simulink model "Autopilot"  (R2025a)
settings: Solver=FixedStepDiscrete  StartTime=0.0  StopTime=600  FixedStep=0.008333  RelTol=1e-3
libraries: slpidlib x2
settings Model: Creator=HP  LastModifiedBy=HP
settings DataIOCC: SaveOutput=off  StreamToWks=off  SaveTime=off  ReturnWorkspaceOutputs=off

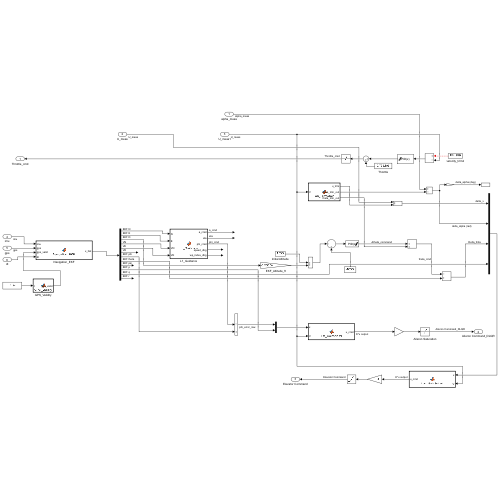
[thumbnail: Simulink's stored preview of the top-level diagram]
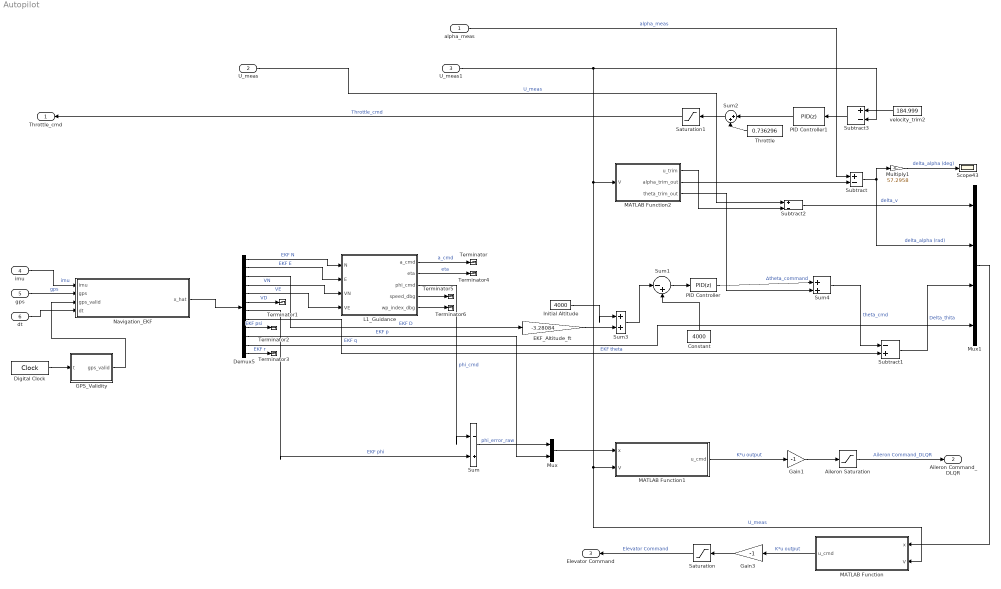
== system Autopilot ==
  alpha_meas : Inport  OutDataTypeStr=double  PortDimensions=1  SampleTime=[0.0083330000000000001,0]
  U_meas : Inport  Port=2  OutDataTypeStr=double  PortDimensions=1  SampleTime=[0.0083330000000000001,0]
  U_meas1 : Inport  Port=3  OutDataTypeStr=double  PortDimensions=1  SampleTime=[0.0083330000000000001,0]
  imu : Inport  Port=4  OutDataTypeStr=double  PortDimensions=[6 1]  SampleTime=[0.0083330000000000001,0]
  gps : Inport  Port=5  OutDataTypeStr=double  PortDimensions=[3 1]  SampleTime=[0.0083330000000000001,0]
  dt : Inport  Port=6  OutDataTypeStr=double  PortDimensions=1  SampleTime=[0.0083330000000000001,0]
  Aileron Saturation : Saturate  UpperLimit=1  LowerLimit=-1
  Constant : Constant  Value=4000  SampleTime=0.008333
  Demux5 : Demux  Outputs=12
  Digital Clock : DigitalClock  SampleTime=0.008333
  EKF_Altitude_ft : Gain  Gain=-3.28084
  GPS_Validity : MATLAB Function  TreatAsAtomicUnit=on  SystemSampleTime=0.008333
  Gain1 : Gain  Gain=-1
  Gain3 : Gain  Gain=-1
  Initial Altitude : Constant  Value=4000  SampleTime=0.008333
  L1_Guidance : MATLAB Function  TreatAsAtomicUnit=on  SystemSampleTime=0.008333
  MATLAB Function : MATLAB Function  TreatAsAtomicUnit=on  SystemSampleTime=0.008333
  MATLAB Function1 : MATLAB Function  TreatAsAtomicUnit=on  SystemSampleTime=0.008333
  MATLAB Function2 : MATLAB Function  TreatAsAtomicUnit=on
  Multiply1 : Gain  Gain=57.2958
  Mux : Mux  Inputs=2
  Mux1 : Mux
  Navigation_EKF : MATLAB Function  TreatAsAtomicUnit=on  SystemSampleTime=0.008333
  PID Controller : slpidlib/PID Controller  Controller=PID  Form=Parallel  TimeDomain=Discrete-time  UseExternalTs=off  SampleTime=0.008333  IntegratorMethod=Forward Euler  FilterMethod=Forward Euler  ControllerParametersSource=internal  P=0.01  I=0.00001  UseKiTs=off  D=0.01  UseExternalDerivativeSource=off  N=115.919945582358  UseFilter=on  TunerSelectOption=Transfer Function Based (PID Tuner App)  InitialConditionSource=internal  InitialConditionForIntegrator=0  InitialConditionForFilter=0  DifferentiatorICPrevScaledInput=0  ExternalReset=none  TrackingMode=off  Kt=1  LimitOutput=on  SatLimitsSource=internal  UpperSaturationLimit=0.2618  LowerSaturationLimit=-0.1745  LinearizeAsGain=on  AntiWindupMode=clamping  Kb=1  LimitIntegrator=off  UpperIntegratorSaturationLimit=inf  LowerIntegratorSaturationLimit=-inf  POutMin=[]  POutMax=[]  IOutMin=[]  IOutMax=[]  DOutMin=[]  DOutMax=[]  NOutMin=[]  NOutMax=[]  SumOutMin=[]  SumOutMax=[]  SaturationOutMin=[]  SaturationOutMax=[]  PParamMin=[]  PParamMax=[]  IParamMin=[]  IParamMax=[]  DParamMin=[]  DParamMax=[]  NParamMin=[]  NParamMax=[]  KbParamMin=[]  KbParamMax=[]  KtParamMin=[]  KtParamMax=[]  KbOutMin=[]  KbOutMax=[]  KtOutMin=[]  KtOutMax=[]  IntegratorOutMin=[]  IntegratorOutMax=[]  FilterOutMin=[]  FilterOutMax=[]  SumI1OutMin=[]  SumI1OutMax=[]  SumI2OutMin=[]  SumI2OutMax=[]  SumI3OutMin=[]  SumI3OutMax=[]  SumI4OutMin=[]  SumI4OutMax=[]  SumDOutMin=[]  SumDOutMax=[]  DifferentiatorOutMin=[]  DifferentiatorOutMax=[]  FilterDiffOutCoefMin=[]  FilterDiffOutCoefMax=[]  ReciprocalOutMin=[]  ReciprocalOutMax=[]  SumDenOutMin=[]  SumDenOutMax=[]  SumNumOutMin=[]  SumNumOutMax=[]  DivideOutMin=[]  DivideOutMax=[]  UdiffTsProdOutMin=[]  UdiffTsProdOutMax=[]  NTsProdOutMin=[]  NTsProdOutMax=[]  UintegralTsProdOutMin=[]  UintegralTsProdOutMax=[]  UngainTsProdOutMin=[]  UngainTsProdOutMax=[]  ClampingZeroOutDataTypeStr=Inherit: Inherit via back propagation  ClampingZeroOutMin=[]  ClampingZeroOutMax=[]  FilterDenConstantOutDataTypeStr=Inherit: Inherit via back propagation  FilterDenConstantOutMin=[]  FilterDenConstantOutMax=[]  PCopyOutDataTypeStr=Inherit: Inherit via back propagation  PCopyOutMin=[]  PCopyOutMax=[]  NCopyOutDataTypeStr=Inherit: Inherit via back propagation  NCopyOutMin=[]  NCopyOutMax=[]  IntegratorContinuousStateAttributes=''  IntegratorStateMustResolveToSignalObject=off  IntegratorRTWStateStorageClass=Auto  FilterContinuousStateAttributes=''  FilterStateMustResolveToSignalObject=off  FilterRTWStateStorageClass=Auto  ParallelPVariant=InternalParameters  IdealPVariant=Disabled  IVariant=InternalParameters  DVariant=InternalParameters  IntegratorVariant=Discrete  SatVariant=Enabled  AWVariant=DiscClampingParallel  PCopyVariant=Disabled  TRVariant=Disabled  FdbkBlocksVariant=Forward  IdealPFdbkVariant=Disabled  SatFdbkVariant=Disabled  DerivativeFilterVariant=ForwardEulerFilter  NVariant=InternalParameters  NCopyVariant=Disabled  FilterICVariant=InternalICsFilter  IntegratorICVariant=InternalICs  ExternalResetVariant=Disabled  TRSumVariant=Passthrough  SumFdbkVariant=Disabled  SumVariant=Sum_PID  TsampFilterVariant=InternalTs  TsampNgainVariant=Passthrough  TsampIntegralVariant=Disabled_SignalSpec  ExternalSaturationOutDataTypeStr=Inherit: Same as second input  DerivativeSourceVariant=ErrorSignal  PreIntVariant=InternalPreInt
  PID Controller1 : slpidlib/PID Controller  Controller=PID  Form=Parallel  TimeDomain=Discrete-time  UseExternalTs=off  SampleTime=0.008333  IntegratorMethod=Forward Euler  FilterMethod=Forward Euler  ControllerParametersSource=internal  P=0.01  I=0.001  UseKiTs=off  D=0  UseExternalDerivativeSource=off  N=100  UseFilter=on  TunerSelectOption=Transfer Function Based (PID Tuner App)  InitialConditionSource=internal  InitialConditionForIntegrator=0  InitialConditionForFilter=0  DifferentiatorICPrevScaledInput=0  ExternalReset=none  TrackingMode=off  Kt=1  LimitOutput=on  SatLimitsSource=internal  UpperSaturationLimit=+0.26  LowerSaturationLimit=-0.73  LinearizeAsGain=on  AntiWindupMode=clamping  Kb=1  LimitIntegrator=off  UpperIntegratorSaturationLimit=inf  LowerIntegratorSaturationLimit=-inf  POutMin=[]  POutMax=[]  IOutMin=[]  IOutMax=[]  DOutMin=[]  DOutMax=[]  NOutMin=[]  NOutMax=[]  SumOutMin=[]  SumOutMax=[]  SaturationOutMin=[]  SaturationOutMax=[]  PParamMin=[]  PParamMax=[]  IParamMin=[]  IParamMax=[]  DParamMin=[]  DParamMax=[]  NParamMin=[]  NParamMax=[]  KbParamMin=[]  KbParamMax=[]  KtParamMin=[]  KtParamMax=[]  KbOutMin=[]  KbOutMax=[]  KtOutMin=[]  KtOutMax=[]  IntegratorOutMin=[]  IntegratorOutMax=[]  FilterOutMin=[]  FilterOutMax=[]  SumI1OutMin=[]  SumI1OutMax=[]  SumI2OutMin=[]  SumI2OutMax=[]  SumI3OutMin=[]  SumI3OutMax=[]  SumI4OutMin=[]  SumI4OutMax=[]  SumDOutMin=[]  SumDOutMax=[]  DifferentiatorOutMin=[]  DifferentiatorOutMax=[]  FilterDiffOutCoefMin=[]  FilterDiffOutCoefMax=[]  ReciprocalOutMin=[]  ReciprocalOutMax=[]  SumDenOutMin=[]  SumDenOutMax=[]  SumNumOutMin=[]  SumNumOutMax=[]  DivideOutMin=[]  DivideOutMax=[]  UdiffTsProdOutMin=[]  UdiffTsProdOutMax=[]  NTsProdOutMin=[]  NTsProdOutMax=[]  UintegralTsProdOutMin=[]  UintegralTsProdOutMax=[]  UngainTsProdOutMin=[]  UngainTsProdOutMax=[]  ClampingZeroOutDataTypeStr=Inherit: Inherit via back propagation  ClampingZeroOutMin=[]  ClampingZeroOutMax=[]  FilterDenConstantOutDataTypeStr=Inherit: Inherit via back propagation  FilterDenConstantOutMin=[]  FilterDenConstantOutMax=[]  PCopyOutDataTypeStr=Inherit: Inherit via back propagation  PCopyOutMin=[]  PCopyOutMax=[]  NCopyOutDataTypeStr=Inherit: Inherit via back propagation  NCopyOutMin=[]  NCopyOutMax=[]  IntegratorContinuousStateAttributes=''  IntegratorStateMustResolveToSignalObject=off  IntegratorRTWStateStorageClass=Auto  FilterContinuousStateAttributes=''  FilterStateMustResolveToSignalObject=off  FilterRTWStateStorageClass=Auto  ParallelPVariant=InternalParameters  IdealPVariant=Disabled  IVariant=InternalParameters  DVariant=InternalParameters  IntegratorVariant=Discrete  SatVariant=Enabled  AWVariant=DiscClampingParallel  PCopyVariant=Disabled  TRVariant=Disabled  FdbkBlocksVariant=Forward  IdealPFdbkVariant=Disabled  SatFdbkVariant=Disabled  DerivativeFilterVariant=ForwardEulerFilter  NVariant=InternalParameters  NCopyVariant=Disabled  FilterICVariant=InternalICsFilter  IntegratorICVariant=InternalICs  ExternalResetVariant=Disabled  TRSumVariant=Passthrough  SumFdbkVariant=Disabled  SumVariant=Sum_PID  TsampFilterVariant=InternalTs  TsampNgainVariant=Passthrough  TsampIntegralVariant=Disabled_SignalSpec  ExternalSaturationOutDataTypeStr=Inherit: Same as second input  DerivativeSourceVariant=ErrorSignal  PreIntVariant=InternalPreInt
  Saturation : Saturate  UpperLimit=1  LowerLimit=-1
  Saturation1 : Saturate  UpperLimit=1  LowerLimit=0
  Scope43 : Scope
      settings: ActiveDisplayYMinimum=-224.04099957405427  ActiveDisplayYMaximum=224.59880182616257  DataLoggingVariableName=ScopeData19
  Subtract : Sum  Inputs=+-
  Subtract1 : Sum  Inputs=-+
  Subtract2 : Sum  Inputs=+-
  Subtract3 : Sum  Inputs=+-
  Sum : Sum  Inputs=|-+
  Sum1 : Sum  Inputs=|-+
  Sum2 : Sum  Inputs=|++
  Sum3 : Sum  Inputs=|++
  Sum4 : Sum  Inputs=|++
  Terminator{,1..6} (7 alike) : Terminator
  Throttle : Constant  Value=0.736296  SampleTime=0.008333
  velocity_trim2 : Constant  Value=184.999  SampleTime=0.008333
  Throttle_cmd : Outport  OutDataTypeStr=double  PortDimensions=1  SampleTime=[0.0083330000000000001,0]
  Aileron Command_DLQR : Outport  Port=2  OutDataTypeStr=double  PortDimensions=1  SampleTime=[0.0083330000000000001,0]
  Elevator Command : Outport  Port=3  OutDataTypeStr=double  PortDimensions=1  SampleTime=[0.0083330000000000001,0]
  wires:
  Multiply1/1 -> Scope43/1  "delta_alpha (deg)"
  Demux5/10 -> Mux/2  "EKF p"
  velocity_trim2/1 -> Subtract3/1
  U_meas1/1 -> MATLAB Function2/1(V), MATLAB Function1/2(V), MATLAB Function/2(V), Subtract3/2  "U_meas"
  Sum3/1 -> Sum1/1
  L1_Guidance/3(phi_cmd) -> Sum/1  "phi_cmd"
  U_meas/1 -> Subtract2/1  "U_meas"
  Gain1/1 -> Aileron Saturation/1
  PID Controller1/1 -> Sum2/1
  Digital Clock/1 -> GPS_Validity/1(t)
  Constant/1 -> Sum1/2
  Demux5/11 -> Mux1/4  "EKF q"
  Initial Altitude/1 -> Sum3/1
  L1_Guidance/5(wp_index_dbg) -> Terminator6/1
  Aileron Saturation/1 -> Aileron Command_DLQR/1  "Aileron Command_DLQR"
  alpha_meas/1 -> Subtract/1  "alpha_meas"
  MATLAB Function1/1(u_cmd) -> Gain1/1  "K*u output"
  Demux5/5 -> L1_Guidance/4(VE)  "VE"
  L1_Guidance/1(a_cmd) -> Terminator/1  "a_cmd"
  Demux5/6 -> Terminator1/1  "VD"
  Navigation_EKF/1(x_hat) -> Demux5/1
  MATLAB Function2/3(theta_trim_out) -> Sum4/2
  imu/1 -> Navigation_EKF/1(imu)  "imu"
  Subtract1/1 -> Mux1/3  "Delta_thita"
  Demux5/9 -> Terminator2/1  "EKF psi"
  MATLAB Function2/1(u_trim) -> Subtract2/2
  Mux/1 -> MATLAB Function1/1(x)
  Sum4/1 -> Subtract1/1  "theta_cmd"
  L1_Guidance/4(speed_dbg) -> Terminator5/1
  Saturation1/1 -> Throttle_cmd/1  "Throttle_cmd"
  PID Controller/1 -> Sum4/1  "Δtheta_command"
  Saturation/1 -> Elevator Command/1  "Elevator Command"
  MATLAB Function/1(u_cmd) -> Gain3/1  "K*u output"
  gps/1 -> Navigation_EKF/2(gps)  "gps"
  L1_Guidance/2(eta) -> Terminator4/1  "eta"
  Demux5/4 -> L1_Guidance/3(VN)  "VN"
  Sum1/1 -> PID Controller/1
  Sum2/1 -> Saturation1/1
  Demux5/2 -> L1_Guidance/2(E)  "EKF E"
  MATLAB Function2/2(alpha_trim_out) -> Subtract/2
  Demux5/1 -> L1_Guidance/1(N)  "EKF N"
  dt/1 -> Navigation_EKF/4(dt)
  Subtract/1 -> Mux1/2, Multiply1/1  "delta_alpha (rad)"
  Gain3/1 -> Saturation/1
  Demux5/12 -> Terminator3/1  "EKF r"
  EKF_Altitude_ft/1 -> Sum3/2
  Mux1/1 -> MATLAB Function/1(x)
  Throttle/1 -> Sum2/2
  Subtract2/1 -> Mux1/1  "delta_v"
  GPS_Validity/1(gps_valid) -> Navigation_EKF/3(gps_valid)
  Subtract3/1 -> PID Controller1/1
  Demux5/7 -> Sum/2  "EKF phi"
  Demux5/8 -> Subtract1/2  "EKF theta"
  Demux5/3 -> EKF_Altitude_ft/1  "EKF D"
  Sum/1 -> Mux/1  "phi_error_raw"

== matlab function Autopilot/MATLAB Function2 ==
  data: V input; u_trim output; alpha_trim_out output; theta_trim_out output
function [u_trim, alpha_trim_out, theta_trim_out] = Lon_TrimSched(V)
V_pts          = [100, 184.999, 220];
u_trim_pts     = [100, 184.999, 220];      % trim speed = design speed, by definition
alpha_trim_pts = [0.148036, 0.00265563, -0.0161908];
theta_trim_pts = [0.148036, 0.00265571, -0.0161907];

u_trim         = interp1(V_pts, u_trim_pts, V, 'linear', 'extrap');
alpha_trim_out = interp1(V_pts, alpha_trim_pts, V, 'linear', 'extrap');
theta_trim_out = interp1(V_pts, theta_trim_pts, V, 'linear', 'extrap');
end

== matlab function Autopilot/Navigation_EKF ==
  data: imu input; x_hat output; gps input; gps_valid input; dt input
function x_hat = Navigation_EKF(imu, gps, gps_valid, dt)
%#codegen
%
% 12-State INS/GPS/Gyro EKF
%
% State:
% x = [N E D VN VE VD phi theta psi p q r]'
%
% IMU:
% imu = [ax ay az p q r]'
%
% GPS:
% gps = [N E D]'
%
% p,q,r are estimated states using the gyro measurements.

GRAVITY = 9.80665;

% =========================================================
% PERSISTENT STATE
% =========================================================

persistent x P initialized

if isempty(initialized)

    x = zeros(12,1);

    % Position from first GPS measurement
    x(1) = gps(1);
    x(2) = gps(2);
    x(3) = gps(3);

    % Initial aircraft velocity
    V0 = 56.4;
    psi0 = deg2rad(225.0);

    x(4) = V0*cos(psi0);
    x(5) = V0*sin(psi0);
    x(6) = 0.0;

    % Initial attitude
    x(7) = 0.0;
    x(8) = 0.0026556;
    x(9) = psi0;

    % Initial body rates from first gyro measurement
    x(10) = imu(4);
    x(11) = imu(5);
    x(12) = imu(6);

    P = diag([ ...
        5.0^2;
        5.0^2;
        5.0^2;
        2.0^2;
        2.0^2;
        2.0^2;
        deg2rad(5.0)^2;
        deg2rad(5.0)^2;
        deg2rad(8.0)^2;
        0.01^2;
        0.01^2;
        0.01^2 ]);

    initialized = true;
end


% =========================================================
% IMU
% =========================================================

ax = imu(1);
ay = imu(2);
az = imu(3);

p = imu(4);
q = imu(5);
r = imu(6);


% =========================================================
% STATE
% =========================================================

phi   = x(7);
theta = x(8);
psi   = x(9);


% =========================================================
% BODY -> NED ROTATION
% =========================================================

cp = cos(phi);
sp = sin(phi);

ct = cos(theta);
st = sin(theta);

cy = cos(psi);
sy = sin(psi);

C_bn = [ ...
    ct*cy, ...
    sp*st*cy - cp*sy, ...
    cp*st*cy + sp*sy;

    ct*sy, ...
    sp*st*sy + cp*cy, ...
    cp*st*sy - sp*cy;

    -st, ...
    sp*ct, ...
    cp*ct ];


% =========================================================
% SPECIFIC FORCE -> NED ACCELERATION
% =========================================================

f_body = [ax; ay; az];

gravity_ned = [0; 0; GRAVITY];

acceleration_ned = C_bn*f_body + gravity_ned;


% =========================================================
% ATTITUDE RATES
% =========================================================

tan_theta = tan(theta);

phi_dot = ...
    p + sp*tan_theta*q + cp*tan_theta*r;

theta_dot = ...
    cp*q - sp*r;

psi_dot = ...
    (sp*q + cp*r)/ct;


% =========================================================
% NONLINEAR STATE DERIVATIVE
% =========================================================

f = zeros(12,1);

f(1) = x(4);
f(2) = x(5);
f(3) = x(6);

f(4) = acceleration_ned(1);
f(5) = acceleration_ned(2);
f(6) = acceleration_ned(3);

f(7) = phi_dot;
f(8) = theta_dot;
f(9) = psi_dot;

% Body rates:
% random-walk model; gyro measurements correct them
f(10) = 0.0;
f(11) = 0.0;
f(12) = 0.0;


% =========================================================
% STATE PREDICTION
% =========================================================

x_pred = x + f*dt;

x_pred(7:9) = ...
    mod(x_pred(7:9) + pi,2*pi) - pi;


% =========================================================
% CONTINUOUS JACOBIAN
% =========================================================

tt = tan(theta);
sec2 = 1.0/(ct*ct);

Fc = zeros(12,12);

% Position
Fc(1,4) = 1.0;
Fc(2,5) = 1.0;
Fc(3,6) = 1.0;


% North acceleration

daN_dphi = ...
    (cp*st*cy + sp*sy)*ay ...
    + (-sp*st*cy + cp*sy)*az;

daN_dtheta = ...
    -st*cy*ax ...
    + sp*ct*cy*ay ...
    + cp*ct*cy*az;

daN_dpsi = ...
    -ct*sy*ax ...
    + (-sp*st*sy - cp*cy)*ay ...
    + (-cp*st*sy + sp*cy)*az;


% East acceleration

daE_dphi = ...
    (cp*st*sy - sp*cy)*ay ...
    + (-sp*st*sy - cp*cy)*az;

daE_dtheta = ...
    -st*sy*ax ...
    + sp*ct*sy*ay ...
    + cp*ct*sy*az;

daE_dpsi = ...
    ct*cy*ax ...
    + (sp*st*cy - cp*sy)*ay ...
    + (cp*st*cy + sp*sy)*az;


% Down acceleration

daD_dphi = ...
    cp*ct*ay ...
    - sp*ct*az;

daD_dtheta = ...
    -ct*ax ...
    - sp*st*ay ...
    - cp*st*az;


Fc(4,7) = daN_dphi;
Fc(4,8) = daN_dtheta;
Fc(4,9) = daN_dpsi;

Fc(5,7) = daE_dphi;
Fc(5,8) = daE_dtheta;
Fc(5,9) = daE_dpsi;

Fc(6,7) = daD_dphi;
Fc(6,8) = daD_dtheta;


% Attitude derivatives

Fc(7,7) = ...
    cp*tt*q - sp*tt*r;

Fc(7,8) = ...
    (sp*q + cp*r)*sec2;

Fc(8,7) = ...
    -sp*q - cp*r;

Fc(9,7) = ...
    (cp*q - sp*r)/ct;

Fc(9,8) = ...
    (sp*q + cp*r)*sec2/ct;


% =========================================================
% DISCRETE TRANSITION
% =========================================================

Fd = eye(12) + Fc*dt;


% =========================================================
% PROCESS NOISE
% =========================================================

Q = diag([ ...
    0.001^2;
    0.001^2;
    0.001^2;
    0.04^2;
    0.04^2;
    0.04^2;
    deg2rad(0.03)^2;
    deg2rad(0.03)^2;
    deg2rad(0.03)^2;
    0.005^2;
    0.005^2;
    0.005^2 ]);


% =========================================================
% COVARIANCE PREDICTION
% =========================================================

P_pred = Fd*P*Fd' + Q;

P_pred = 0.5*(P_pred + P_pred');


% =========================================================
% MEASUREMENT MODEL
%
% z = [GPS_N GPS_E GPS_D gyro_p gyro_q gyro_r]'
% =========================================================

H = zeros(6,12);

H(1,1) = 1.0;
H(2,2) = 1.0;
H(3,3) = 1.0;

H(4,10) = 1.0;
H(5,11) = 1.0;
H(6,12) = 1.0;


z = [ ...
    gps(1);
    gps(2);
    gps(3);
    p;
    q;
    r ];


z_pred = H*x_pred;

innovation = z - z_pred;


% =========================================================
% MEASUREMENT NOISE
% =========================================================

R = diag([ ...
    2.0^2;
    2.0^2;
    3.0^2;
    0.002^2;
    0.002^2;
    0.002^2 ]);


% =========================================================
% GPS VALIDITY
%
% If GPS is unavailable, ignore the first 3 measurements.
% Gyro measurements remain active.
% =========================================================

if gps_valid == 0

    H_use = H(4:6,:);
    z_use = z(4:6);
    z_pred_use = z_pred(4:6);
    R_use = R(4:6,4:6);

    innovation_use = z_use - z_pred_use;

    S = H_use*P_pred*H_use' + R_use;

    K = P_pred*H_use'/S;

    x = x_pred + K*innovation_use;

    I12 = eye(12);
    A = I12 - K*H_use;

    P = A*P_pred*A' + K*R_use*K';

else

    S = H*P_pred*H' + R;

    K = P_pred*H'/S;

    x = x_pred + K*innovation;

    I12 = eye(12);
    A = I12 - K*H;

    P = A*P_pred*A' + K*R*K';

end


% =========================================================
% COVARIANCE SYMMETRY
% =========================================================

P = 0.5*(P + P');


% =========================================================
% ANGLE WRAP
% =========================================================

x(7:9) = ...
    mod(x(7:9) + pi,2*pi) - pi;


% =========================================================
% OUTPUT
% =========================================================

x_hat = x;

end

== matlab function Autopilot/GPS_Validity ==
  data: t input; gps_valid output
function gps_valid = GPS_Validity(t)
if t >= 25.0 && t < 35.0
    gps_valid = 0;
else
    gps_valid = 1;
end






%gps_valid = 1; % TEMP forced on -- see README, revert before final submission
% Original outage logic (restore after this test):
% if t >= 25.0 && t < 35.0
%     gps_valid = 0;
% else
%     gps_valid = 1;
% end

== matlab function Autopilot/L1_Guidance ==
  data: N input; a_cmd output; eta output; E input; VN input; VE input; phi_cmd output; speed_dbg output; wp_index_dbg output
function [a_cmd, eta, phi_cmd, speed_dbg, wp_index_dbg] = L1_Guidance(N, E, VN, VE)
%#codegen
%
% ============================================================
% C172P — FOUR-WAYPOINT CLOSED-PATH L1 GUIDANCE
% ============================================================
%
% Fixed-wing autonomous path following
%
% Navigation convention:
%   North = +N
%   East  = +E
%x
% Inputs:
%   N  = EKF North position [m]
%   E  = EKF East position  [m]
%   VN = EKF North velocity [m/s]
%   VE = EKF East velocity  [m/s]
%
% Outputs:
%   a_cmd   = commanded lateral acceleration [m/s^2]
%   eta     = L1 guidance angle [rad]
%   phi_cmd = commanded bank angle [rad]
%
% DEBUG OUTPUTS (added for WP2/WP4 S-wiggle speed-coupling diagnosis --
% not part of the guidance law, safe to remove once the diagnostic
% run is done):
%   speed_dbg    = current EKF horizontal ground speed [m/s]
%   wp_index_dbg = active waypoint index (1-4), as double for logging
%
% Architecture:
%
%       EKF
%        |
%        v
%   L1 Guidance
%        |
%        v
%     phi_cmd
%        |
%        v
%   existing DLQR
%        |
%        v
%     Aileron
%        |
%        v
%      C172P
%
% ============================================================
% GUIDANCE LAW
% ============================================================
%
% Standard L1 lateral acceleration law:
%
%       a_cmd = 2*V^2/L1_dist*sin(eta)
%
% where:
%
%       V = current horizontal ground-speed magnitude
%
%       V = sqrt(VN^2 + VE^2)
%
% IMPORTANT:
%
% The L1 guidance law uses the CURRENT EKF velocity.
%
% The nominal aircraft trim speed is:
%
%       185.0 ft/s  (TRUE airspeed / ground speed, no-wind assumption)
%       = 56.388 m/s
%
% but this is NOT hard-coded into the L1 guidance law.
%
% The aircraft may accelerate/decelerate during turns,
% climbs, transients, and other manoeuvres. L1 therefore
% uses the instantaneous estimated horizontal velocity.
%
% ============================================================
% PATH MANAGEMENT
% ============================================================
%
% Closed four-waypoint path with automatic waypoint switching.
%
% Waypoints:
%
%       WP1 = (-4500, -4500)
%       WP2 = (    0, -9000)
%       WP3 = ( 4500, -4500)
%       WP4 = (    0,     0)
%
% Segment sequence:
%
%       WP4 -> WP1 : 225 deg
%       WP1 -> WP2 : 135 deg
%       WP2 -> WP3 :  45 deg
%       WP3 -> WP4 : 315 deg
%
% Each corner is approximately a 90-degree turn.
%
% ============================================================


% ============================================================
% CONSTANTS
% ============================================================

g = 9.80665;

% Nominal C172P cruise trim speed.
%
% This value is documented here for traceability only.
% It is NOT used directly in the L1 calculation.
%
% CORRECTED: use TRUE airspeed (= ground speed, no-wind), not
% calibrated airspeed. speed = sqrt(VN^2+VE^2) below is computed
% from EKF ground-referenced velocity, so the traceability constant
% must use the same physical quantity: 185.0 ft/s true, not the
% 174.426 ft/s calibrated-airspeed reading JSBSim reports for the
% same trim condition at 4000 ft. Mixing the two here previously
% understated phi_max by about 0.9 deg.
%
% 185.0 ft/s = 56.388 m/s

V_trim_nominal = 185.0 * 0.3048;

% L1 lookahead distance [m]
L1_dist = 350.0;

% Maximum bank command, set to the standard-rate-turn bank angle
% (3 deg/sec turn rate) at the nominal trim speed:
%
%       phi_std = atan(V * omega_std / g)
%       V        = 56.388 m/s   (185.0 ft/s TRUE trim speed)
%       omega_std= 3 deg/s      (standard rate, aviation convention)
%       phi_std  = atan(56.388 * deg2rad(3) / 9.80665)
%                ≈ 16.76 deg
%
% Original value (7 deg) was too shallow for this waypoint geometry:
% turn radius at 7 deg exceeds half the waypoint leg length, so the
% aircraft never straightens out between corners (see gain-scheduling
% session notes / README). A second correction (this one) fixed the
% derivation itself: the original 16 deg was computed from calibrated
% airspeed (174.426 ft/s) instead of the true/ground speed (185 ft/s)
% that the live guidance law actually uses. 17 deg is the corrected
% standard-rate-turn value, rounded to a clean, citable number the
% same way the original 16 deg was.
%
% IMPORTANT:
% phi_max is a bank-angle limit. The L1 acceleration command
% itself is generated from the current aircraft speed.

phi_max = deg2rad(17.0);

% Waypoint acceptance radius [m]
%
% This is NOT the L1 lookahead distance.
% It determines when the active waypoint is considered reached.

waypoint_radius = 350.0;


% ============================================================
% FOUR CLOSED-PATH WAYPOINTS
% ============================================================

WP1_N = -4500.0;
WP1_E = -4500.0;

WP2_N =     0.0;
WP2_E = -9000.0;

WP3_N =  4500.0;
WP3_E = -4500.0;

WP4_N =     0.0;
WP4_E =     0.0;


% ============================================================
% PERSISTENT ACTIVE-WAYPOINT STATE
% ============================================================
%
% waypoint_index:
%
%       1 -> WP1
%       2 -> WP2
%       3 -> WP3
%       4 -> WP4
%
% After WP4, the path closes back to WP1.

persistent waypoint_index

if isempty(waypoint_index)
    waypoint_index = int32(1);
end


% ============================================================
% CURRENT AIRCRAFT SPEED
% ============================================================
%
% IMPORTANT:
%
% Use instantaneous EKF horizontal velocity.
%
% Do NOT replace this with V_trim_nominal.
%
% V_trim_nominal is only the nominal design/traceability value.

speed = sqrt( ...
    VN*VN + ...
    VE*VE);


if speed < 1e-6

    a_cmd = 0.0;
    eta = 0.0;
    phi_cmd = 0.0;
    speed_dbg = speed;
    wp_index_dbg = double(waypoint_index);

    return;

end


% ============================================================
% VEHICLE VELOCITY UNIT VECTOR
% ============================================================

vel_dir_N = VN / speed;
vel_dir_E = VE / speed;


% ============================================================
% CURRENT ACTIVE PATH SEGMENT
% ============================================================

if waypoint_index == 1

    start_N = WP4_N;
    start_E = WP4_E;

    end_N = WP1_N;
    end_E = WP1_E;

elseif waypoint_index == 2

    start_N = WP1_N;
    start_E = WP1_E;

    end_N = WP2_N;
    end_E = WP2_E;

elseif waypoint_index == 3

    start_N = WP2_N;
    start_E = WP2_E;

    end_N = WP3_N;
    end_E = WP3_E;

else

    start_N = WP3_N;
    start_E = WP3_E;

    end_N = WP4_N;
    end_E = WP4_E;

end


% ============================================================
% CHECK DISTANCE TO ACTIVE WAYPOINT
% ============================================================

distance_to_waypoint = sqrt( ...
    (N - end_N)*(N - end_N) + ...
    (E - end_E)*(E - end_E));


if distance_to_waypoint < waypoint_radius

    waypoint_index = waypoint_index + int32(1);

    if waypoint_index > 4
        waypoint_index = int32(1);
    end


    % Re-select the active segment immediately.

    if waypoint_index == 1

        start_N = WP4_N;
        start_E = WP4_E;

        end_N = WP1_N;
        end_E = WP1_E;

    elseif waypoint_index == 2

        start_N = WP1_N;
        start_E = WP1_E;

        end_N = WP2_N;
        end_E = WP2_E;

    elseif waypoint_index == 3

        start_N = WP2_N;
        start_E = WP2_E;

        end_N = WP3_N;
        end_E = WP3_E;

    else

        start_N = WP3_N;
        start_E = WP3_E;

        end_N = WP4_N;
        end_E = WP4_E;

    end

end


% ============================================================
% PATH VECTOR
% ============================================================

path_N = end_N - start_N;
path_E = end_E - start_E;

path_length = sqrt( ...
    path_N*path_N + ...
    path_E*path_E);


if path_length < 1e-6

    a_cmd = 0.0;
    eta = 0.0;
    phi_cmd = 0.0;
    speed_dbg = speed;
    wp_index_dbg = double(waypoint_index);

    return;

end


% ============================================================
% PATH UNIT VECTOR
% ============================================================

path_dir_N = path_N / path_length;
path_dir_E = path_E / path_length;


% ============================================================
% PROJECT AIRCRAFT ONTO ACTIVE PATH
% ============================================================

relative_N = N - start_N;
relative_E = E - start_E;

along_track = ...
    relative_N * path_dir_N + ...
    relative_E * path_dir_E;


% ============================================================
% CONSTRAIN PROJECTION TO ACTIVE SEGMENT
% ============================================================

if along_track < 0.0

    along_track_clamped = 0.0;

elseif along_track > path_length

    along_track_clamped = path_length;

else

    along_track_clamped = along_track;

end


% ============================================================
% L1 LOOKAHEAD POINT
% ============================================================

lookahead_distance = ...
    along_track_clamped + L1_dist;


if lookahead_distance > path_length

    lookahead_distance = path_length;

end


l1_N = ...
    start_N + ...
    lookahead_distance * path_dir_N;


l1_E = ...
    start_E + ...
    lookahead_distance * path_dir_E;


% ============================================================
% VECTOR FROM AIRCRAFT TO L1 POINT
% ============================================================

l1_vector_N = l1_N - N;
l1_vector_E = l1_E - E;

l1_length = sqrt( ...
    l1_vector_N*l1_vector_N + ...
    l1_vector_E*l1_vector_E);


if l1_length < 1e-6

    a_cmd = 0.0;
    eta = 0.0;
    phi_cmd = 0.0;
    speed_dbg = speed;
    wp_index_dbg = double(waypoint_index);

    return;

end


% ============================================================
% L1 VECTOR UNIT VECTOR
% ============================================================

l1_dir_N = l1_vector_N / l1_length;
l1_dir_E = l1_vector_E / l1_length;


% ============================================================
% SIGNED L1 GUIDANCE ANGLE
% ============================================================

cross_value = ...
    vel_dir_N * l1_dir_E ...
    - vel_dir_E * l1_dir_N;


dot_value = ...
    vel_dir_N * l1_dir_N ...
    + vel_dir_E * l1_dir_E;


eta = atan2( ...
    cross_value, ...
    dot_value);


% ============================================================
% STANDARD L1 LATERAL ACCELERATION LAW
% ============================================================
%
%       a_cmd = 2*V^2/L1*sin(eta)
%
% V is the CURRENT aircraft speed.
%
% ============================================================

a_cmd = ...
    2.0 * speed*speed / L1_dist * sin(eta);


% ============================================================
% LATERAL ACCELERATION -> BANK ANGLE
% ============================================================

phi_cmd = atan( ...
    a_cmd / g);


% ============================================================
% BANK ANGLE LIMIT
% ============================================================

if phi_cmd > phi_max

    phi_cmd = phi_max;

elseif phi_cmd < -phi_max

    phi_cmd = -phi_max;

end


% ============================================================
% DEBUG OUTPUTS (normal-path assignment)
% ============================================================

speed_dbg = speed;
wp_index_dbg = double(waypoint_index);


end

== matlab function Autopilot/MATLAB Function ==
  data: x input; u_cmd output; V input
function u_cmd = Lon_GainSched(x, V)
V_pts = [100, 185, 220];
K_pts = [0.0176, 1.5810, -7.7995, -2.4150;
         0.0213, 2.2732, -7.5064, -2.1186;
         0.0198, 2.3520, -7.1666, -2.0173];
K_now = zeros(1,4);
for i = 1:4
    K_now(i) = interp1(V_pts, K_pts(:,i), V, 'linear', 'extrap');
end
u_cmd = K_now * x;

== matlab function Autopilot/MATLAB Function1 ==
  data: x input; u_cmd output; V input
function u_cmd = Lat_GainSched(x, V)
V_pts = [100, 185, 220];
K_pts = [2.2724, 0.6695;
         2.2368, 0.5453;
         2.2149, 0.5334];
K_now = zeros(1,2);
for i = 1:2
    K_now(i) = interp1(V_pts, K_pts(:,i), V, 'linear', 'extrap');
end
u_cmd = K_now * x;
